simulink model "LCK_DanishV01"  (R2018b)
settings: Solver=FixedStepDiscrete  StartTime=0.0  StopTime=inf  FixedStep=0.01  RelTol=1e-3
PostLoadFcn:
  | if any(exist('dsrtsu_mdlpostloadfcn', 'file') ~= 0), dsrtsu_mdlpostloadfcn('Execute', bdroot); end
values from neighbouring files (symbols this model uses):
  C_DEG2RAD = 0.0175    [LCK_Macro.sldd]
  C_KPH2MPS = 0.2778    [LCK_Macro.sldd]
  C_NEARZERO = 0.0001    [LCK_Macro.sldd]
  C_ONE = 1.0    [LCK_Macro.sldd]
  C_RAD2DEG = 57.2958    [LCK_Macro.sldd]
  C_ZERO = 0.0    [LCK_Macro.sldd]
  k_accel_pedal_pos_per_speed_x : value not decoded    [LCK_LogicPara.sldd]
  k_accel_pedal_pos_per_speed_z : value not decoded    [LCK_LogicPara.sldd]
  k_brake_suprress_hold = 1000.0    [LCK_LogicPara.sldd]
  k_driver_appl_torque_filt = 50.0    [LCK_LogicPara.sldd]
  k_driver_suppression_hold_time = 3000.0    [LCK_LogicPara.sldd]
  k_hands_on_wheel_hold_msec = 500.0    [LCK_LogicPara.sldd]
  k_hands_on_wheel_torque_hi = 0.2    [LCK_LogicPara.sldd]
  k_hands_on_wheel_torque_lo = 0.15    [LCK_LogicPara.sldd]
  k_handsoff_delay_cycles = 50.0    [LCK_LogicPara.sldd]
  k_handsoff_torq_Lo_CR = 0.3    [LCK_LogicPara.sldd]
  k_handson_delay_cycles = 5.0    [LCK_LogicPara.sldd]
  k_HighAccel_suppress_hold = 3000.0    [LCK_LogicPara.sldd]
  k_HLR_suprress_hold = 3000.0    [LCK_LogicPara.sldd]
  k_hs_StrAng_CR_threshold_z : value not decoded    [LCK_LogicPara.sldd]
  k_LC_Exit_Switch = 0.0    [LCK_LogicPara.sldd]
  k_LCG_Configured = 1.0    [LCK_LogicPara.sldd]
  k_LCK_A0_Rdy2Act_UseConst = 0.0    [LCK_LogicPara.sldd]
  k_LCK_A0Fac_ActSta : value not decoded    [LCK_CtrlPara.sldd]
  k_LCK_A0Fac_DrvStm : value not decoded    [LCK_CtrlPara.sldd]
  k_LCK_A0Shift_LftCurv : value not decoded    [LCK_CtrlPara.sldd]
  k_LCK_A0Shift_RgtCurv : value not decoded    [LCK_CtrlPara.sldd]
  k_LCK_A0Shift_StraLan = 0.0    [LCK_CtrlPara.sldd]
  k_LCK_A0ShiftFac_Dy_LftCurv : value not decoded    [LCK_CtrlPara.sldd]
  k_LCK_A0ShiftFac_Dy_RgtCurv : value not decoded    [LCK_CtrlPara.sldd]
  k_LCK_A0ShiftFac_Vspd : value not decoded    [LCK_CtrlPara.sldd]
  k_LCK_accel_inhibit_thold = 35.0    [LCK_LogicPara.sldd]
  k_LCK_Active2Ready_Mask = 255.0    [LCK_LogicPara.sldd]
  k_LCK_CvatRateBks : value not decoded    [LCK_CtrlPara.sldd]
  k_LCK_CvatrBks : value not decoded    [LCK_CtrlPara.sldd]
  k_LCK_DFac_Dy : value not decoded    [LCK_CtrlPara.sldd]
  k_LCK_DFac_Dy_Curv : value not decoded    [LCK_CtrlPara.sldd]
  k_LCK_DFac_HaCurCen : value not decoded    [LCK_CtrlPara.sldd]
  k_LCK_DFac_HaCurSid : value not decoded    [LCK_CtrlPara.sldd]
  k_LCK_DFac_HadCurCen : value not decoded    [LCK_CtrlPara.sldd]
  k_LCK_DFac_HadCurSid : value not decoded    [LCK_CtrlPara.sldd]
  k_LCK_DFac_HadStrCen : value not decoded    [LCK_CtrlPara.sldd]
  k_LCK_DFac_HadStrSid : value not decoded    [LCK_CtrlPara.sldd]
  k_LCK_DFac_HaStrCen : value not decoded    [LCK_CtrlPara.sldd]
  k_LCK_DFac_HaStrSid : value not decoded    [LCK_CtrlPara.sldd]
  k_LCK_DFac_Rad : value not decoded    [LCK_CtrlPara.sldd]
  k_LCK_DFac_SA_CurCen : value not decoded    [LCK_CtrlPara.sldd]
  k_LCK_DFac_SA_CurSid : value not decoded    [LCK_CtrlPara.sldd]
  k_LCK_DFac_SA_StrCen : value not decoded    [LCK_CtrlPara.sldd]
  k_LCK_DFac_SA_StrSid : value not decoded    [LCK_CtrlPara.sldd]
  k_LCK_DFac_SS_CurCen : value not decoded    [LCK_CtrlPara.sldd]
  k_LCK_DFac_SS_CurSid : value not decoded    [LCK_CtrlPara.sldd]
  k_LCK_DFac_SS_StrCen : value not decoded    [LCK_CtrlPara.sldd]
  k_LCK_DFac_SS_StrSid : value not decoded    [LCK_CtrlPara.sldd]
  k_LCK_DFac_Vspd : value not decoded    [LCK_CtrlPara.sldd]
  k_LCK_DlyTm_DrvStim = 0.2    [LCK_CtrlPara.sldd]
  k_LCK_DTermMax = 2.0    [LCK_CtrlPara.sldd]
  k_LCK_DyBks_Curv : value not decoded    [LCK_CtrlPara.sldd]
  k_LCK_Enable_POOnly = 1.0    [LCK_LogicPara.sldd]
  k_LCK_Entry_DistBuffer = 0.1    [LCK_LogicPara.sldd]
  k_LCK_Fac_Vspd2RngThr_FalRec = 0.23    [LCK_CtrlPara.sldd]
  k_LCK_Ffw_CvatSwh = 0.0    [LCK_CtrlPara.sldd]
  k_LCK_Ffw_DyBks : value not decoded    [LCK_CtrlPara.sldd]
  k_LCK_Ffw_TimCon_CmdFlt = 0.0    [LCK_CtrlPara.sldd]
  k_LCK_FfwDeltaFac_Rad_Lft : value not decoded    [LCK_CtrlPara.sldd]
  k_LCK_FfwDeltaFac_Rad_Rgt : value not decoded    [LCK_CtrlPara.sldd]
  k_LCK_FfwDeltaFac_Vspd : value not decoded    [LCK_CtrlPara.sldd]
  k_LCK_FfwFac_CvatRate_Lft : value not decoded    [LCK_CtrlPara.sldd]
  k_LCK_FfwFac_CvatRate_Rgt : value not decoded    [LCK_CtrlPara.sldd]
  k_LCK_FfwFac_Dy : value not decoded    [LCK_CtrlPara.sldd]
  k_LCK_FfwFac_Rad_Lft : value not decoded    [LCK_CtrlPara.sldd]
  k_LCK_FfwFac_Rad_Rgt : value not decoded    [LCK_CtrlPara.sldd]
  k_LCK_FfwFac_Vspd : value not decoded    [LCK_CtrlPara.sldd]
  k_LCK_FfwTorq_Cvat : value not decoded    [LCK_CtrlPara.sldd]
  k_LCK_HAFac_ActSta : value not decoded    [LCK_CtrlPara.sldd]
  k_LCK_HAFac_DrvStm : value not decoded    [LCK_CtrlPara.sldd]
  k_LCK_HaloTime = 2000.0    [LCK_LogicPara.sldd]
  k_LCK_HaloTime_Switch = 0.0    [LCK_LogicPara.sldd]
  k_LCK_HARFac_ActSta : value not decoded    [LCK_CtrlPara.sldd]
  k_LCK_HARFac_DrvStm : value not decoded    [LCK_CtrlPara.sldd]
  k_LCK_Hed_DyBks : value not decoded    [LCK_CtrlPara.sldd]
  k_LCK_HedAngDiffX : value not decoded    [LCK_CtrlPara.sldd]
  k_LCK_HedAngRateDiffX : value not decoded    [LCK_CtrlPara.sldd]
  k_LCK_HndsOnWhel_DlyTm_Idl2Rdy = 0.0    [LCK_LogicPara.sldd]
  k_LCK_host_veh_width = 1.86    [LCK_LogicPara.sldd]
  k_LCK_Idle2Ready_Mask = 239.0    [LCK_LogicPara.sldd]
  k_LCK_Junc_SusTime = 1.0    [LCK_LogicPara.sldd]
  k_LCK_KpKdDecSlopeLmt = 10.0    [LCK_CtrlPara.sldd]
  k_LCK_KpKdIncSlopeLmt = 5.0    [LCK_CtrlPara.sldd]
  k_LCK_Lat_Ctrl_DFac_Lft = 1.0    [LCK_CtrlPara.sldd]
  k_LCK_Lat_Ctrl_DFac_Rgt = 1.05    [LCK_CtrlPara.sldd]
  k_LCK_Lat_Ctrl_Kd = 0.8    [LCK_CtrlPara.sldd]
  k_LCK_Lat_Ctrl_Ki = 0.5    [LCK_CtrlPara.sldd]
  k_LCK_Lat_Ctrl_Kp = 0.7    [LCK_CtrlPara.sldd]
  k_LCK_Lat_Ctrl_Kp_NearGain = 0.7    [LCK_CtrlPara.sldd]
  k_LCK_Lat_Ctrl_PFac_Lft = 1.0    [LCK_CtrlPara.sldd]
  k_LCK_Lat_Ctrl_PFac_Rgt = 1.05    [LCK_CtrlPara.sldd]
  k_LCK_Lat_Ctrl_TimCon_CmdFlt = 5.0    [LCK_CtrlPara.sldd]
  k_LCK_Lat_DFac_Rad : value not decoded    [LCK_CtrlPara.sldd]
  k_LCK_Lat_DFac_SS_Cur : value not decoded    [LCK_CtrlPara.sldd]
  k_LCK_Lat_DFac_SS_Str : value not decoded    [LCK_CtrlPara.sldd]
  k_LCK_Lat_DFac_Vspd : value not decoded    [LCK_CtrlPara.sldd]
  k_LCK_Lat_DyBks : value not decoded    [LCK_CtrlPara.sldd]
  k_LCK_Lat_IFac_Rad : value not decoded    [LCK_CtrlPara.sldd]
  k_LCK_Lat_IFac_Vspd : value not decoded    [LCK_CtrlPara.sldd]
  k_LCK_Lat_ILmtFac_Dy_CurvLan : value not decoded    [LCK_CtrlPara.sldd]
  k_LCK_Lat_ILmtFac_Dy_StraLan : value not decoded    [LCK_CtrlPara.sldd]
  k_LCK_Lat_ILmtFac_Rad : value not decoded    [LCK_CtrlPara.sldd]
  k_LCK_Lat_ILmtFac_Rad_NearGain = 1.0    [LCK_CtrlPara.sldd]
  k_LCK_Lat_ILmtFac_Vspd_CurvLan : value not decoded    [LCK_CtrlPara.sldd]
  k_LCK_Lat_ILmtFac_Vspd_StraLan : value not decoded    [LCK_CtrlPara.sldd]
  k_LCK_Lat_ITermLmt_Dy = 1.0    [LCK_CtrlPara.sldd]
  k_LCK_Lat_KpKdDecSlopeLmt = 10.0    [LCK_CtrlPara.sldd]
  k_LCK_Lat_KpKdIncSlopeLmt = 10.0    [LCK_CtrlPara.sldd]
  k_LCK_Lat_PFac_Dy_InnLftCur : value not decoded    [LCK_CtrlPara.sldd]
  k_LCK_Lat_PFac_Dy_InnRgtCur : value not decoded    [LCK_CtrlPara.sldd]
  k_LCK_Lat_PFac_Dy_OutLftCur : value not decoded    [LCK_CtrlPara.sldd]
  k_LCK_Lat_PFac_Dy_OutRgtCur : value not decoded    [LCK_CtrlPara.sldd]
  k_LCK_Lat_PFac_Dy_Str : value not decoded    [LCK_CtrlPara.sldd]
  k_LCK_Lat_PFac_Rad : value not decoded    [LCK_CtrlPara.sldd]
  ... (+153 more)
undefined symbols (not defined in the file or in its folder): k_LCK_CurvBks, K_LCK_SPA0A1A2_LMRngCmp_y
libraries: LateralControl_fcns_lib x58, simulink x24
(part 8 of 47)

== system LCK_DanishV01/Lateral_Control_Module/Adas_Lateral_Control_LCK_Core/Module 10 ==
  Vspd : Inport
  Dy_0 : Inport  Port=2
  Curvature_0 : Inport  Port=3
  Curvature_1 : Inport  Port=4
  Curvat_Rate : Inport  Port=5
  Road_Radius : Inport  Port=6
  Bus Creator8 : BusCreator  Inputs=5
  Calculation of Feed Forward Torq : Subsystem
  First_Order_Lag_Filter_LIB : LateralControl_fcns_lib/First_Order_Lag_Filter_LIB  SystemSampleTime=-1
  Gain{,1..3} (4 alike) : Gain
  ML_TIME_MSEC2 : Constant  Description=_GWMAB30P3.LCK.000_166_  Value=ML_TIME_MSEC
  k_LCK_Ffw_TimCon_CmdFlt : Constant  Description=_GWMAB30P3.LCK.000_168_  Value=k_LCK_Ffw_TimCon_CmdFlt
  Ffw_Ctrl_Info : Outport
  wires:
  k_LCK_Ffw_TimCon_CmdFlt/1 -> First_Order_Lag_Filter_LIB/2
  ML_TIME_MSEC2/1 -> First_Order_Lag_Filter_LIB/3
  First_Order_Lag_Filter_LIB/1 -> Bus Creator8/5  "Ffw_Ctrl_Cmd"
  Calculation of Feed Forward Torq/5(Feed_Forward_Torq) -> First_Order_Lag_Filter_LIB/1
  Vspd/1 -> Calculation of Feed Forward Torq/1(Vspd)
  Dy_0/1 -> Calculation of Feed Forward Torq/2(Current_Dy)
  Curvat_Rate/1 -> Calculation of Feed Forward Torq/3(Curvat_Rat)
  Curvature_0/1 -> Calculation of Feed Forward Torq/4(Curvature_0)
  Curvature_1/1 -> Calculation of Feed Forward Torq/5(Curvature_1)
  Road_Radius/1 -> Calculation of Feed Forward Torq/6(Road_Radius)
  Calculation of Feed Forward Torq/4(FfwTorq_Delta) -> Gain3/1
  Calculation of Feed Forward Torq/1(FfwFac_CvatRate) -> Gain1/1
  Bus Creator8/1 -> Ffw_Ctrl_Info/1
  Calculation of Feed Forward Torq/2(FfwFac_Dy) -> Gain/1
  Calculation of Feed Forward Torq/3(FfwTorq_Basic) -> Gain2/1
  Gain1/1 -> Bus Creator8/1
  Gain/1 -> Bus Creator8/2
  Gain2/1 -> Bus Creator8/3
  Gain3/1 -> Bus Creator8/4

== system LCK_DanishV01/Lateral_Control_Module/Adas_Lateral_Control_LCK_Core/Module 11 ==
  Lat_Ctrl_Cmd : Inport
  LatCtrl_Cmd : Inport  Port=2
  Ffw_Ctrl_Cmd : Inport  Port=3
  SPP_Recognition_Type : Inport  Port=4
  Vspd : Inport  Port=5
  Lat_Ctrl_State : Inport  Description=_GWMAB30P4.LCK.000_293_  Port=6
  Bus Creator : BusCreator  Inputs=3
  Non-Linear Compenastion : Subsystem
  Terminator : Terminator
  Torque_Cmd_Rate_Limit : Subsystem
  LCK_FinalTorqCmd : Outport
  wires:
  [Vspd] -> Torque_Cmd_Rate_Limit/3(Vspd)
  Vspd/1 -> Non-Linear Compenastion/5(Vspd), [Vspd]
  Lat_Ctrl_Cmd/1 -> Non-Linear Compenastion/1(Lat_Ctrl_Cmd)
  LatCtrl_Cmd/1 -> Non-Linear Compenastion/2(LatCtrl_Cmd)
  Ffw_Ctrl_Cmd/1 -> Non-Linear Compenastion/3(Ffw_Ctrl_Cmd)
  Torque_Cmd_Rate_Limit/1(TorqCmd_RateLimited) -> LCK_FinalTorqCmd/1
  Lat_Ctrl_State/1 -> Torque_Cmd_Rate_Limit/2(Lat_Ctrl_State)
  Non-Linear Compenastion/1(LCK_PIDTorqCmd) -> Bus Creator/1  "LCK_PID_TorqCmd"
  Non-Linear Compenastion/2(LCK_PIDPlusFfw_TorqCmd) -> Bus Creator/2  "LCK_PIDPlusFfw_TorqCmd"
  SPP_Recognition_Type/1 -> Non-Linear Compenastion/4(SPPRecognition_Type)
  Non-Linear Compenastion/3(LCK_PIDTorqCmd_Percent) -> Bus Creator/3  "LCK_PIDTorqCmd_Percent"
  Bus Creator/1 -> Terminator/1
  Non-Linear Compenastion/4(LCK_TorqCmd_Cmpd) -> Torque_Cmd_Rate_Limit/1(TorqCmd)

== system LCK_DanishV01/Lateral_Control_Module/Adas_Lateral_Control_LCK_Core/Module 12 ==
  Lat_Ctrl_State : Inport
  LC_Info : Inport  Port=2
  SPP_Coeff : Inport  Port=3
  Bus Selector1 : BusSelector  OutputSignals=SPP_A0_Fltd
  Bus Selector2 : BusSelector  OutputSignals=LC_A1
  Bus Selector3 : BusSelector  OutputSignals=LC_A0
  Bus Selector4 : BusSelector  OutputSignals=SPP_A1_Fltd
  Bus Selector5 : BusSelector  OutputSignals=LC_A2
  Bus Selector6 : BusSelector  OutputSignals=SPP_A2_Fltd
  Bus Selector7 : BusSelector  OutputSignals=SPP_A3_Fltd
  Constant2 : Constant  Tag={'output',{'name','$P','class','EXTERN_MACRO','type','ESR_Typedefs/unsigned8_T'},'date',737462.69417376153}  Description=_GWMH9P4.LCK.000_202_  OutDataTypeStr=uint8
  Relational Operator3 : RelationalOperator  Operator=>  OutDataTypeStr=boolean  RndMeth=Nearest
  Switch1 : Switch  Description=_GWMAB30P2.LCK.000_1368_  Threshold=0.5
  Switch10 : Switch  Description=_GWMAB30P2.LCK.000_1368_  Threshold=0.5
  Switch2 : Switch  Description=_GWMAB30P2.LCK.000_1368_  Threshold=0.5
  Trj_A0 : Outport  Description=_GWMH9P3.LCK.000_786_
  Trj_A1 : Outport  Description=_GWMH9P3.LCK.000_786_  Port=2
  Trj_A2 : Outport  Description=_GWMH9P3.LCK.000_786_  Port=3
  Trj_A3 : Outport  Description=_GWMH9P3.LCK.000_786_  Port=4
  wires:
  Constant2/1 -> Relational Operator3/2
  Lat_Ctrl_State/1 -> Relational Operator3/1
  Relational Operator3/1 -> Switch10/2, Switch2/2, Switch1/2
  LC_Info/1 -> Bus Selector5/1, Bus Selector2/1, Bus Selector3/1
  Bus Selector3/1 -> Switch10/1  "<LC_A0>"
  SPP_Coeff/1 -> Bus Selector7/1, Bus Selector6/1, Bus Selector4/1, Bus Selector1/1
  Bus Selector1/1 -> Switch10/3  "<SPP_A0_Fltd>"
  Switch10/1 -> Trj_A0/1
  Bus Selector2/1 -> Switch1/1  "<LC_A1>"
  Bus Selector4/1 -> Switch1/3  "<SPP_A1_Fltd>"
  Bus Selector5/1 -> Switch2/1  "<LC_A2>"
  Bus Selector6/1 -> Switch2/3  "<SPP_A2_Fltd>"
  Switch1/1 -> Trj_A1/1
  Switch2/1 -> Trj_A2/1
  Bus Selector7/1 -> Trj_A3/1  "<SPP_A3_Fltd>"

== system LCK_DanishV01/Lateral_Control_Module/Adas_Lateral_Control_LCK_Core/Module 2 ==
  Vspd : Inport
  IMU_Yaw_Rt_Pri : Inport  Port=2
  Road_Radius : Inport  Port=3
  Curvature_0 : Inport  Port=4
  Str_Flag : Inport  Port=5
  Cur_Flag : Inport  Port=6
  SPP_A0 : Inport  Port=7
  Calculation of Heading Angle Rate : Subsystem
  Constant25 : Constant  Tag={'output',{'name','$P','class','EXTERN_MACRO','type','ESR_Typedefs/unsigned8_T'},'date',737462.69417376153}  Description=_GWMH9P4.LCK.000_202_  Value=ML_TIME_MSEC
  First_Order_Lag_Filter_LIB : LateralControl_fcns_lib/First_Order_Lag_Filter_LIB  SystemSampleTime=-1
  k_LCK_TimCon_YawRtFlt : Constant  Tag={'output',{'name','$P','class','EXTERN_CAL','type','Float32'},'date',737503.54997206014}  Description=_GACA26P3.LCK.000_83_  Value=k_LCK_TimCon_YawRtFlt
  Hed_Ang_Rat : Outport
  wires:
  Calculation of Heading Angle Rate/1(Hed_Ang_Rat) -> Hed_Ang_Rat/1
  Constant25/1 -> First_Order_Lag_Filter_LIB/3
  k_LCK_TimCon_YawRtFlt/1 -> First_Order_Lag_Filter_LIB/2
  First_Order_Lag_Filter_LIB/1 -> Calculation of Heading Angle Rate/1(Yaw_Rate)
  Road_Radius/1 -> Calculation of Heading Angle Rate/2(Road_Radius)
  Curvature_0/1 -> Calculation of Heading Angle Rate/3(Curvature_0)
  Vspd/1 -> Calculation of Heading Angle Rate/4(Vspd)
  IMU_Yaw_Rt_Pri/1 -> First_Order_Lag_Filter_LIB/1
  SPP_A0/1 -> Calculation of Heading Angle Rate/5(SPP_A0)
  Str_Flag/1 -> Calculation of Heading Angle Rate/6(Str_Flag)
  Cur_Flag/1 -> Calculation of Heading Angle Rate/7(Cur_Flag)

== system LCK_DanishV01/Lateral_Control_Module/Adas_Lateral_Control_LCK_Core/Module 3 ==
  Lat_Ctrl_State : Inport
  Steer_Torq : Inport  Port=2
  Bus Creator3 : BusCreator  Inputs=2
  Determination_Sig_Wekng_Factor : Subsystem
  Sig_Wekng_0 : Subsystem
  Sig_Wekng_1 : Subsystem
  Sig_Wekng_Factor : Outport
  Sig_Wekng_Flag : Outport  Port=2
  wires:
  Steer_Torq/1 -> Sig_Wekng_1/1(Steer_Torq)
  Lat_Ctrl_State/1 -> Sig_Wekng_0/1(Lat_Ctrl_State)
  Determination_Sig_Wekng_Factor/1(Sig_Wekng_Factor) -> Sig_Wekng_Factor/1
  Sig_Wekng_0/1(A0Fac_ActSta) -> Determination_Sig_Wekng_Factor/1(A0Fac_ActSta)
  Sig_Wekng_1/4(HARFac_DrvStm) -> Determination_Sig_Wekng_Factor/6(HARFac_DrvStm)
  Sig_Wekng_0/2(HAFac_ActSta) -> Determination_Sig_Wekng_Factor/2(HAFac_ActSta)
  Sig_Wekng_1/2(A0Fac_DrvStm) -> Determination_Sig_Wekng_Factor/4(A0Fac_DrvStm)
  Sig_Wekng_1/3(HAFac_DrvStm) -> Determination_Sig_Wekng_Factor/5(HAFac_DrvStm)
  Sig_Wekng_0/3(HARFac_ActSta) -> Determination_Sig_Wekng_Factor/3(HARFac_ActSta)
  Sig_Wekng_0/4(Act_Start_Falg_Held) -> Bus Creator3/1  "Act_Start_Falg_Held"
  Sig_Wekng_1/1(Drv_Stm_Flag_Held) -> Bus Creator3/2  "Drv_Stm_Flag_Held"
  Bus Creator3/1 -> Sig_Wekng_Flag/1
